simulink model "half_bridge_NPC_inverter"  (R2021a)
settings: Solver=ode4  StartTime=0.0  StopTime=0.1  FixedStep=1e-6  RelTol=1e-3
libraries: spsIGBTDiodeLib x4, spsDCVoltageSourceLib x2, spsDiodeLib x2, spsGroundLib x2, simulink x2, spsVoltageMeasurementLib x1, spspowerguiLib x1
settings Model: Creator=PRANAY KAMAL  LastModifiedBy=PRANAY KAMAL
settings DataIOCC: ReturnWorkspaceOutputs=off

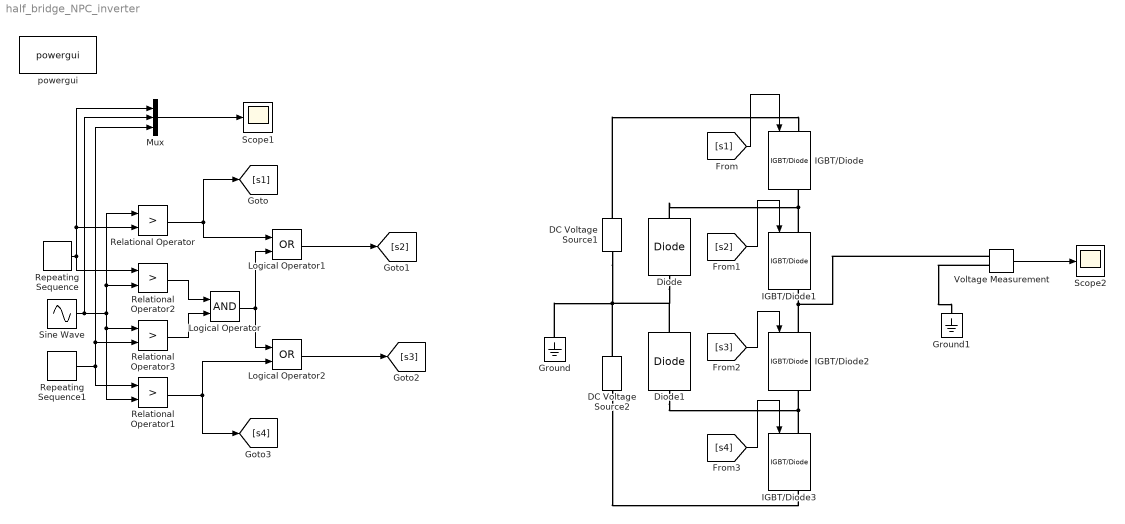
== system half_bridge_NPC_inverter ==
  DC Voltage Source1 : spsDCVoltageSourceLib/DC Voltage Source  Amplitude=200  Measurements=None
  DC Voltage Source2 : spsDCVoltageSourceLib/DC Voltage Source  Amplitude=200  Measurements=None
  Diode : spsDiodeLib/Diode  Ron=0.001  Lon=0  Vf=0.8  IC=0  UseSnubber=0  Rs=500  Cs=250e-9  Measurements=off
  Diode1 : spsDiodeLib/Diode  Ron=0.001  Lon=0  Vf=0.8  IC=0  UseSnubber=0  Rs=500  Cs=250e-9  Measurements=off
  Ground : spsGroundLib/Ground  LConnTagsString=a
  Ground1 : spsGroundLib/Ground  LConnTagsString=a
  IGBT/Diode{,1..3} (4 alike) : spsIGBTDiodeLib/IGBT//Diode  Ron=1e-3  Rs=1e5  Cs=inf  Measurements=on
  Logical Operator : Logic  AllPortsSameDT=off  OutDataTypeStr=boolean
  Logical Operator1 : Logic  Operator=OR  AllPortsSameDT=off  OutDataTypeStr=boolean
  Logical Operator2 : Logic  Operator=OR  AllPortsSameDT=off  OutDataTypeStr=boolean
  Mux : Mux  Inputs=3
  Relational Operator{,1..3} (4 alike) : RelationalOperator  Operator=>  OutDataTypeStr=boolean  RndMeth=Simplest
  Repeating Sequence : simulink/Sources/Repeating Sequence  rep_seq_t=[0 0.5 1]*(1/6000)  rep_seq_y=[1 0 1]
  Repeating Sequence1 : simulink/Sources/Repeating Sequence  rep_seq_t=[0 0.5 1]*(1/6000)  rep_seq_y=[0 -1 0]
  Scope1 : Scope
  Scope2 : Scope
  Sine Wave : Sin  Amplitude=0.8  Frequency=2*pi*60  SampleTime=0
  Voltage Measurement : spsVoltageMeasurementLib/Voltage Measurement  PhasorSimulation=off  OutputType=Complex  PSBequivalent=0
  powergui : spspowerguiLib/powergui  Priority=1  SimulationMode=Continuous  SampleTime=50e-6  frequency=60  Iterations=50  frequencyindice=0  Pbase=100e6  ErrMax=1e-4  UnitsV=kV  UnitsW=MW  buscounter=0  FunctionMessages=off  echomessages=off  EnableUseOfTLC=off  CurrentSourceSwitches=off  DisableSnubberDevices=off  DisableRonSwitches=off  DisableVfSwitches=off  DisplayEquations=off  AutomaticDiscreteSolvers=off  SolverType=Tustin/Backward Euler (TBE)  Interpol=off  ExternalGateDelay=off  methode=off  Ts=100  x0status=blocks  SPID=on  SwTol=0  HookPort=off  NonlinearTolerance=1e-4  nMaxIteration=100  ContinueOnMaxIteration=off  RestoreLinks=warning  ResistiveCurrentMeasurement=off  Frange=[0:2:500]  Ylog=off  Xlog=on  ShowGrid=off  save=off  variable=ZData  structure=0  ZoomFFT=off  StartTime=0.0  cycles=1  DisplayStyle=1  fundamental=60  FreqAxis=off  MaxFrequency=1000  frequencyindicesteady=1  RmsSteady=1  display=off
  wires:
  Sine Wave/1 -> Mux/2, Relational Operator1/2, Relational Operator3/1, Relational Operator2/2, Relational Operator/1
  Repeating Sequence/1 -> Relational Operator2/1, Mux/1, Relational Operator/2
  Repeating Sequence1/1 -> Relational Operator1/1, Relational Operator3/2, Mux/3
  [s1] -> IGBT/Diode/1
  [s2] -> IGBT/Diode1/1
  [s3] -> IGBT/Diode2/1
  [s4] -> IGBT/Diode3/1
  Mux/1 -> Scope1/1
  Voltage Measurement/1 -> Scope2/1
  Relational Operator2/1 -> Logical Operator/1
  Relational Operator3/1 -> Logical Operator/2
  Relational Operator/1 -> Logical Operator1/1, [s1]
  Relational Operator1/1 -> [s4], Logical Operator2/2
  Logical Operator1/1 -> [s2]
  Logical Operator/1 -> Logical Operator2/1, Logical Operator1/2
  Logical Operator2/1 -> [s3]
  connections:
  IGBT/Diode1/LConn1 -- Diode/RConn1 -- IGBT/Diode/RConn1
  IGBT/Diode2/LConn1 -- Voltage Measurement/LConn1 -- IGBT/Diode1/RConn1
  IGBT/Diode3/LConn1 -- Diode1/LConn1 -- IGBT/Diode2/RConn1
  DC Voltage Source1/RConn1 -- IGBT/Diode/LConn1
  DC Voltage Source2/LConn1 -- IGBT/Diode3/RConn1
  Voltage Measurement/LConn2 -- Ground1/LConn1
  Diode1/RConn1 -- Diode/LConn1 -- DC Voltage Source2/RConn1 -- DC Voltage Source1/LConn1 -- Ground/LConn1
